simulink model "gstut12"  (Simulink 6.0)
settings: Solver=FixedStepDiscrete  StartTime=0.0  StopTime=0.5  RelTol=1e-3
undefined symbols (not defined in the file or in its folder): get, hot
libraries: dspbuff3 x2, dspsnks4 x2, dspspect3 x1, dspsrcs4 x1, dspmtrx3 x1, dspmathops x1
settings Model: LastModifiedBy=cclarke
settings DataIOCC: SignalLoggingName=logsOut
settings DebuggingCC: CheckExecutionContextPreStartOutputMsg=on  CheckExecutionContextRuntimeOutputMsg=on
settings ModelReferenceCC: UpdateModelReferenceTargets=IfOutOfDate
settings GRTTargetCC: LifeSpan=inf
settings SFSimCC: SFSimApplyToAllLibs=on  SFSimBuildMode=Incremental

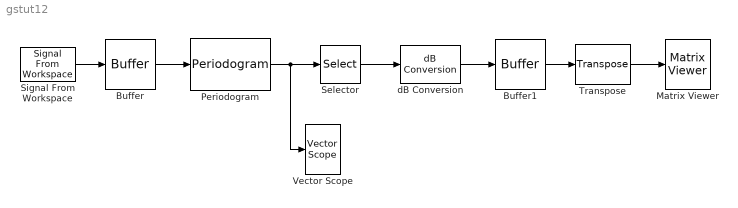
== system gstut12 ==
  Buffer : dspbuff3/Buffer  N=128  V=48  ic=0
  Buffer1 : dspbuff3/Buffer  N=64  V=0  ic=0
  Matrix Viewer : dspsnks4/Matrix Viewer  ImageParams=off  CMapStr=hot(256)  AxisColorbar=on  AxisParams=off  AxisOrigin=Upper left corner  XLabel=X-axis  YLabel=Y-axis  ZLabel=Z-axis  FigPos=get(0,'defaultfigureposition')  AxisZoom=off
      settings: YMin=-1.0  YMax=1.0
  Periodogram : dspspect3/Periodogram  wintype=Hamming  Rs=50  beta=5  winsamp=Periodic  inheritFFT=on  fftsize=256  navg=2
  Selector : Selector  Elements=[1 3]  InputPortWidth=3
  Signal From Workspace : dspsrcs4/Signal From Workspace  X=mtlb  Ts=1/8000  nsamps=80  OutputAfterFinalValue=Setting to zero
  Transpose : dspmtrx3/Transpose  Hermitian=off  overflowFlag=on
  Vector Scope : dspsnks4/Vector Scope  ScopeProperties=on  Domain=Frequency  HorizSpan=1  DisplayProperties=off  AxisGrid=on  Memory=off  FrameNumber=on  AxisLegend=off  AxisZoom=off  OpenScopeAtSimStart=on  OpenScopeImmediately=off  FigPos=get(0,'defaultfigureposition')  AxisProperties=off  XUnits=Hertz  XRange=[0...Fs/2]  InheritXIncr=on  XIncr=1  XLabel=Time  YUnits=dB  YLabel=Magnitude, dB  LineProperties=off
      settings: YMin=-49.3106585941378  YMax=5.11522162658351
  dB Conversion : dspmathops/dB Conversion  dBtype=dB  intype=Amplitude  R=1  fuzz=off
  wires:
  Signal From Workspace/1 -> Buffer/1
  Buffer/1 -> Periodogram/1
  Periodogram/1 -> Vector Scope/1, Selector/1
  Selector/1 -> dB Conversion/1
  dB Conversion/1 -> Buffer1/1
  Buffer1/1 -> Transpose/1
  Transpose/1 -> Matrix Viewer/1
